simulink model "Openloop_Model"  (R2018a)
settings: Solver=VariableStepAuto  StartTime=0.0  StopTime=25  RelTol=1e-3
values from neighbouring files (symbols this model uses):
  b = 0.1    [DC_Motormfile.m]
  JM = 0.4    [DC_Motormfile.m]
  KE = 0.12    [DC_Motormfile.m]    (also in pid.m)
  KT = 0.25    [DC_Motormfile.m]    (also in pid.m)
  L = 493*10^-9    (= 4.93e-07)    [DC_Motormfile.m]    (also in pid.m)
  R = 5.3*10^-3    (= 0.0053)    [DC_Motormfile.m]    (also in pid.m)
  Scaling_Velocity = Sc/(Cw)*Rg*KE    (= 4.865)    [pid.m]
  Ts = 0.01    [pid.m]
settings Model: Creator=MAFAZ  LastModifiedBy=MAFAZ

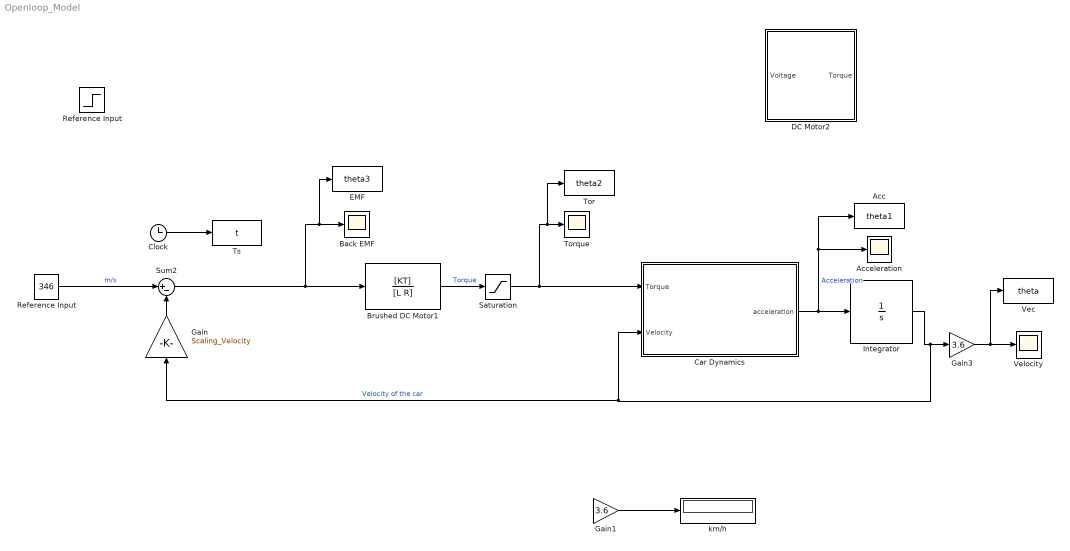
== system Openloop_Model ==
  Acc : ToWorkspace  VariableName=theta1  SampleTime=Ts
  Acceleration : Scope
  Back EMF : Scope
  Brushed DC Motor1 : TransferFcn  Numerator=[KT]  Denominator=[L R]
  Car Dynamics : MATLAB Function  TreatAsAtomicUnit=on
  Clock : Clock
  DC Motor2 : Subsystem
  EMF : ToWorkspace  VariableName=theta3  SampleTime=Ts
  Gain : Gain  Gain=Scaling_Velocity
  Gain1 : Gain  Gain=3.6
  Gain3 : Gain  Gain=3.6
  Integrator : Integrator
  Reference Input : Constant  Value=346
  "Reference Input " : Step  Time=0  After=346  SampleTime=0
  Saturation : Saturate  UpperLimit=600  LowerLimit=0
  Sum2 : Sum  Inputs=|+-
  Tor : ToWorkspace  VariableName=theta2  SampleTime=Ts
  "Torque " : Scope
  Ts : ToWorkspace  VariableName=t  SampleTime=Ts
  Vec : ToWorkspace  VariableName=theta  SampleTime=Ts
  Velocity : Scope
  km/h : Display
  wires:
  Integrator/1 -> Gain/1, Car Dynamics/2(Velocity), Gain3/1  "Velocity of the car"
  Gain3/1 -> Vec/1, Velocity/1
  Gain1/1 -> km/h/1
  Clock/1 -> Ts/1
  Car Dynamics/1(acceleration) -> Acc/1, Acceleration/1, Integrator/1  "Acceleration"
  Reference Input/1 -> Sum2/1  "m/s"
  Gain/1 -> Sum2/2
  Sum2/1 -> EMF/1, Back EMF/1, Brushed DC Motor1/1
  Saturation/1 -> Tor/1, "Torque "/1, Car Dynamics/1(Torque)
  Brushed DC Motor1/1 -> Saturation/1  "Torque"

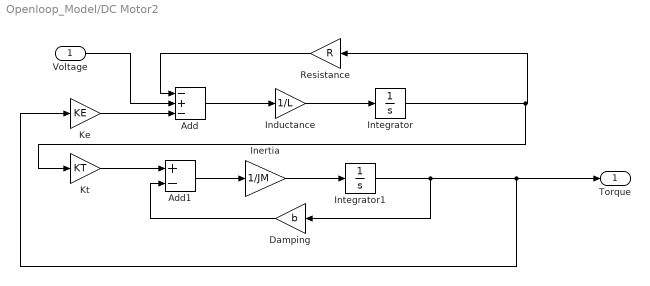
== system Openloop_Model/DC Motor2 ==
  Voltage : Inport
  Add : Sum  Inputs=-+-
  Add1 : Sum  Inputs=+-
  Damping : Gain  Gain=b
  Inductance : Gain  Gain=1/L
  Inertia : Gain  Gain=1/JM
  Integrator : Integrator
  Integrator1 : Integrator
  Ke : Gain  Gain=KE
  Kt : Gain  Gain=KT
  Resistance : Gain  Gain=R
  Torque : Outport
  wires:
  Damping/1 -> Add1/2
  Add1/1 -> Inertia/1
  Integrator/1 -> Kt/1, Resistance/1
  Inertia/1 -> Integrator1/1
  Ke/1 -> Add/3
  Add/1 -> Inductance/1
  Voltage/1 -> Add/2
  Inductance/1 -> Integrator/1
  Integrator1/1 -> Damping/1, Torque/1, Ke/1
  Kt/1 -> Add1/1
  Resistance/1 -> Add/1

== matlab function Openloop_Model/Car Dynamics ==
  data: Torque input; acceleration output; Velocity input
function acceleration = fcn(Torque, Velocity)
acceleration = (40.5*Torque*0.6-413-0.3381*Velocity^2)/2108;

% 0.6 = mechanical efficiency of the vehcile - to ensure its reaches 100
% km/h within 4.4 secs. 

% 413 = actual Rolling Resistance 
%0.3381 = drag force created by the movement of the car

%2108 = mass of the car
